simulink model "jprd"  (R2022b)
settings: Solver=VariableStepAuto  StartTime=0.0  StopTime=100  RelTol=1e-3
libraries: simulink x1
settings Model: Creator=zuzanna  LastModifiedBy=zuzanna

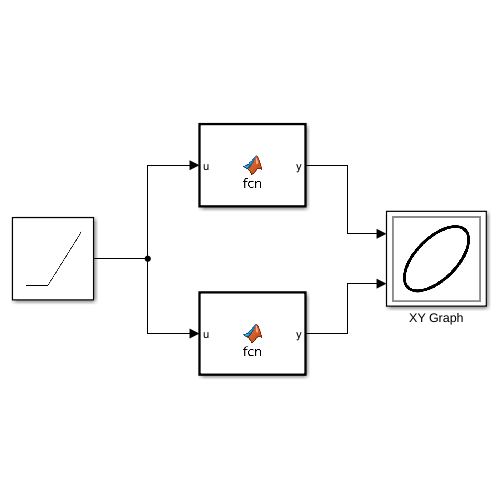
[thumbnail: Simulink's stored preview of the top-level diagram]
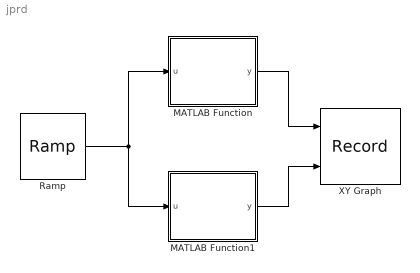
== system jprd ==
  MATLAB Function : MATLAB Function  TreatAsAtomicUnit=on
  MATLAB Function1 : MATLAB Function  TreatAsAtomicUnit=on
  Ramp : simulink/Sources/Ramp  slope=1  start=0  InitialOutput=0
  XY Graph : Record  FileSettingsInternal="{\"entries\":[{\"content\":{\"excelSettings\":{\"content\":{},\"type\":\"Streamout.ExcelSettings\"}},\"type\":\"Streamout.FileSettingStorage\",\"uuid\":\"19814ef5-d199-43e1-a747-a295bd12499e\"}],\"packageUris\":[\"http://schema.mathworks.com/mf0/streamout_blocks/R2020a\"],\"version\":\"1.0\"}"  Layout=[1 1]  SignalsInternal="{\"entries\":[{\"content\":{\"signals\":[{\"content\":{\"blockPath\":[\"jprd/XY Graph\"],\"channel\":[],\"dimensions\":[1],\"domain\":\"jprd/XY Graph\",\"lineColor\":\"#0072bd\",\"plots\":[],\"port\":1,\"sid\":[\"\"],\"signalID\":293,\"signalName\":\"MATLAB Function\"},\"type\":\"RecordBlkView.Signal\",\"uuid\":\"02c4d44d-8dd6-40df-a837-6a17c308e2c1\"},{\"content\":{\"blockPath\":[\"jprd/XY Graph\"],\"channel\":[],\"dimensions\":[1],\"domain\":\"jprd/XY Graph\",\"lineColor\":\"#d95319\",\"plots\":[],\"port\":2,\"sid\":[\"\"],\"signalID\":297,\"signalName\":\"MATLAB Function1\"},\"type\":\"RecordBlkView.Signal\",\"uuid\":\"ce3d4740-a9f9-4fa6-8d1f-6b177e8283d1\"}]},\"type\":\"RecordBlkView.InputSignals\",\"uuid\":\"f78d1b55-3f65-4bb5-ac42-5790ede1067e\"}],\"packageUris\":[\"http://schema.mathworks.com/mf0/streamout_blocks/R2020a\"],\"version\":\"1.0\"}"  VisualizationBindings="{\"xyplotplugin\":{\"info\":[{\"series\":[],\"subplotID\":1}]}}"  CompatibilityTag=XY
  wires:
  Ramp/1 -> MATLAB Function1/1(u), MATLAB Function/1(u)
  MATLAB Function/1(y) -> XY Graph/1
  MATLAB Function1/1(y) -> XY Graph/2

== matlab function jprd/MATLAB Function ==
  data: u input; y output
function y = fcn(u)

y = 1/(1+u^2);

== matlab function jprd/MATLAB Function1 ==
  data: u input; y output
function y = fcn(u)

y = -u/(1+u^2);
